simulink model "threeStateSM"  (R2024b)
settings: Solver=VariableStepAuto  StartTime=0.0  StopTime=10.0  RelTol=1e-3
settings Model: Creator=optimus  LastModifiedBy=optimus

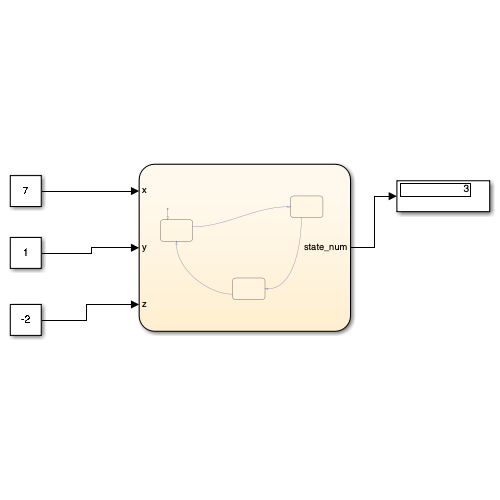
[thumbnail: Simulink's stored preview of the top-level diagram]
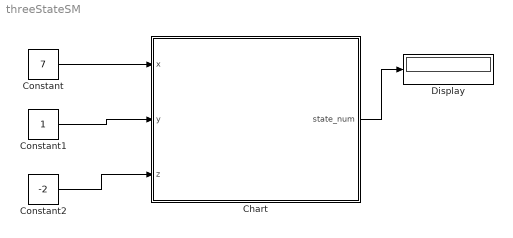
== system threeStateSM ==
  Chart : Stateflow chart  TreatAsAtomicUnit=on
  Constant : Constant  Value=7
  Constant1 : Constant
  Constant2 : Constant  Value=-2
  Display : Display
  wires:
  Chart/1(state_num) -> Display/1
  Constant/1 -> Chart/1(x)
  Constant1/1 -> Chart/2(y)
  Constant2/1 -> Chart/3(z)

== stateflow chart threeStateSM/Chart ==
  state state2
    entry:state_num=2;
  state state1
    entry: state_num=1;
  state state3
    entry:state_num=3;
  state1 -> state2 : [x>5]
  (default) -> state1
  state2 -> state3 : [y==1]
  state3 -> state1 : [z<0]
  data: x input size=1; y input size=1; z input size=1; state_num output size=1
